simulink model "quadrotor_20181106"  (R2016a)
settings: Solver=VariableStepAuto  StartTime=t_0  StopTime=T  MaxStep=MaxStep  RelTol=RelTol  AbsTol=AbsTol
values from neighbouring files (symbols this model uses):
  J = 35000    [initialization.m]
  rule = 1    [initialization.m]
  T = 18    [initialization.m]
  x_0 = [x_0_pre;Lya_0]    [fcn_initial_uniform_eta.m]    (also in initialization.m = x_0_vec(:,i))
libraries: simulink x3
settings Model: Creator=xzbdf  LastModifiedBy=xzbdf

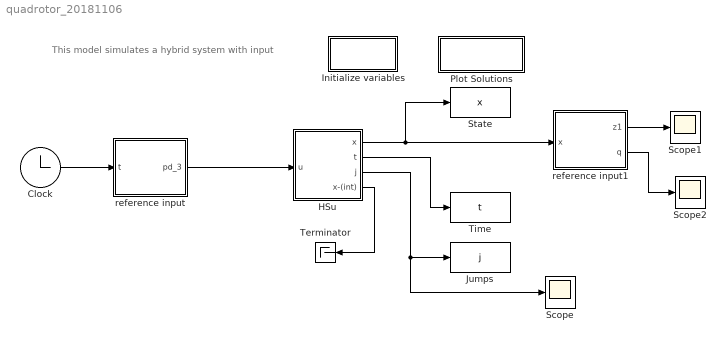
== system quadrotor_20181106 ==
  note: This model simulates a hybrid system with input
  Clock : Clock
  HSu : Subsystem  LoadFcn=set_param(gcb,'LinkStatus','none')
      settings: CopyFcn=|
      | set_param(gcb,'LinkStatus','none'),
      | set_param(gcs, 'MaxStep', 'MaxStep', 'RelTol', 'RelTol','Stop time', 'T')
      mask Display:
      | image(imread('Hcal.jpg'))
      | %plot([5 20 20 5 5],[5 5 20 20 5])
      | %text(8,13,'HyEq_mdl')
      | port_label('output', 1, 'x')
      | port_label('output', 2, 't')
      | port_label('output', 3, 'j')
      | port_label('output', 4, 'x-(int)')
      | port_label('input', 1, 'u')
  Initialize variables : Subsystem  Priority=-10
      settings: OpenFcn=|
      | try
      |      clearvars -except inifile pathfile_in pathfile_pos posfile
      |      cd(pathfile_in);
      |      eval(inifile);
      | catch
      |      [inifile,pathfile_in] = getInitializationfile;
      |      cd(pathfile_in);
      |      inifile = strrep(inifile,'.m','');
      |      eval(inifile);
      | end
      mask Display: disp('Double Click\n to Initialize')
  Jumps : ToWorkspace  VariableName=j  SampleTime=-1
      settings: Save2DSignal=2-D array (concatenate along first dimension)
  Plot Solutions : Subsystem
      settings: OpenFcn=|
      | try
      |      cd(pathfile_pos);
      |      eval(posfile);
      | catch
      |      [posfile,pathfile_pos] = getInitializationfile;
      |      cd(pathfile_pos);
      |      posfile = strrep(posfile,'.m','');
      |      eval(posfile);
      | end
      mask Display: disp('Double Click to\n Plot Solutions')
  Scope : Scope
  Scope1 : Scope
  Scope2 : Scope
  State : ToWorkspace  VariableName=x  SampleTime=-1
  Terminator : Terminator
  Time : ToWorkspace  VariableName=t  SampleTime=-1
      settings: Save2DSignal=2-D array (concatenate along first dimension)
  reference input : MATLAB Function  TreatAsAtomicUnit=on
  reference input1 : MATLAB Function  TreatAsAtomicUnit=on
  wires:
  Clock/1 -> reference input/1(t)
  reference input/1(pd_3) -> HSu/1(u)
  HSu/4(x-(int)) -> Terminator/1
  HSu/1(x) -> reference input1/1(x), State/1
  HSu/2(t) -> Time/1
  HSu/3(j) -> Scope/1, Jumps/1
  reference input1/1(z1) -> Scope1/1
  reference input1/2(q) -> Scope2/1

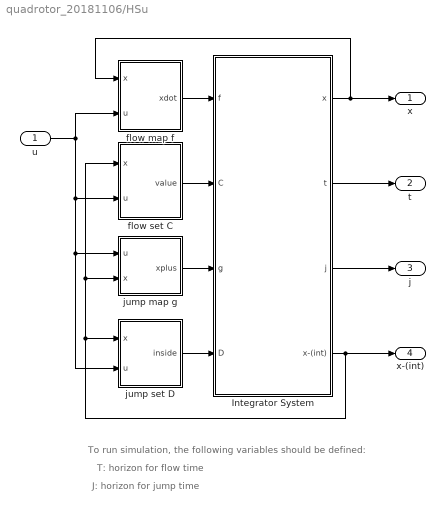
== system quadrotor_20181106/HSu ==
  note: J: horizon for jump time
  note: T: horizon for flow time
  note: To run simulation, the following variables should be defined:
  u : Inport
  Integrator System : Subsystem  Priority=2  mask(Hybrid Integrator){T=T, J=J, x0=x_0}
      mask prompts: T "Flow Horizon"; J "Jump Horizon"; x0 "Initial Condition"
      mask help:
      | This block integrates the state of the hybrid system defined by the flow map f (first input), the flow set C (second input), the jump map g (third input) and the jump set D (fourth input).
      | Starting from the initial condition x0 (last mask parameter), the system's state x evolves continuously within the set C, according to f(x,u), but is also subject to jumps within D, according to g(x,u).
      | The block also stops the simulation when the time t is greater than the flow horizon T (first mask parameter), or when the number of jumps j is greater than the jump horizon J (second mask parameter).
      | The outputs of the blocks are respectively x(t), t, j, x(t-).
      mask Help:
      | This block integrates the state of the hybrid system defined by the flow map f (first input), the flow set C (second input), the jump map g (third input) and the jump set D (fourth input).
      | <br>
      | Starting from the initial condition x0 (last mask parameter), the system's state x evolves continuously within the set C, according to f(x,u), but is also subject to jumps within D, according to g(x,u).
      | <br>
      | The block also stops the simulation when the time t is greater than the flow horizon T (first mask parameter), or when the number of jumps j is greater than the jump horizon J (second mask parameter).
      | <br>
      | The outputs of the blocks are respectively x(t), t, j, x(t-).
      | <br>
      | You can right click on the block and "Look under mask" to see what's inside the block.
      | Finally, refer to the manual (HybridSimulator_vXX.pdf) for more detailed information on how this hybrid simulator works.
  flow map f : MATLAB Function  TreatAsAtomicUnit=on
  flow set C : MATLAB Function  TreatAsAtomicUnit=on
  jump map g : MATLAB Function  Priority=2  TreatAsAtomicUnit=on
  jump set D : MATLAB Function  TreatAsAtomicUnit=on
  x : Outport
  t : Outport  Port=2
  j : Outport  Port=3
  x-(int) : Outport  Port=4
  wires:
  jump map g/1(xplus) -> Integrator System/3(g)
  jump set D/1(inside) -> Integrator System/4(D)
  u/1 -> jump set D/2(u), jump map g/1(u), flow set C/2(u), flow map f/2(u)
  Integrator System/3(j) -> j/1
  Integrator System/2(t) -> t/1
  flow set C/1(value) -> Integrator System/2(C)
  Integrator System/1(x) -> x/1, flow map f/1(x)
  Integrator System/4(x-(int)) -> x-(int)/1, flow set C/1(x), jump map g/2(x), jump set D/1(x)
  flow map f/1(xdot) -> Integrator System/1(f)

== system quadrotor_20181106/Initialize variables ==

== system quadrotor_20181106/Plot Solutions ==

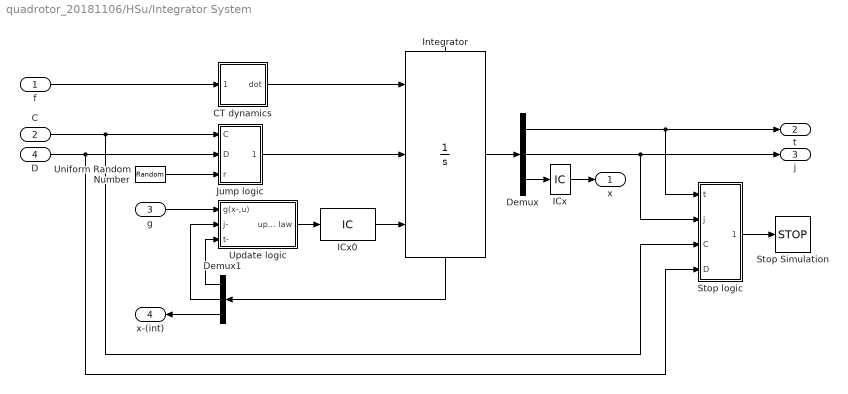
== system quadrotor_20181106/HSu/Integrator System ==
  f : Inport
  C : Inport  Port=2
  g : Inport  Port=3
  D : Inport  Port=4
  CT dynamics : Subsystem
  Demux : Demux  Outputs=[1 1 -1]
  Demux1 : Demux  Outputs=[1 1 -1]
  ICx : InitialCondition  Value=x_0
  ICx0 : InitialCondition  Value=[0; 0; x_0(:)]
  Integrator : Integrator  ExternalReset=level hold  InitialConditionSource=external  ShowStatePort=on  ZeroCross=off
  Jump logic : Subsystem
  Stop Simulation : Stop
  Stop logic : Subsystem
  Uniform Random Number : UniformRandomNumber  Minimum=0  Seed=abs(floor(100*rand))  SampleTime=0
  Update logic : Subsystem
  x : Outport
  t : Outport  Port=2
  j : Outport  Port=3
  x-(int) : Outport  Port=4
  wires:
  ICx0/1 -> Integrator/3
  ICx/1 -> x/1
  Demux/3 -> ICx/1
  Integrator/State -> Demux1/1
  Demux/2 -> j/1, Stop logic/2(j)
  Demux/1 -> t/1, Stop logic/1(t)
  Update logic/1(update law) -> ICx0/1
  CT dynamics/1(dot) -> Integrator/1
  Stop logic/1(stop) -> Stop Simulation/1
  Integrator/1 -> Demux/1
  C/1 -> Stop logic/3(C), Jump logic/1(C)
  D/1 -> Stop logic/4(D), Jump logic/2(D)
  f/1 -> CT dynamics/1(f(x,u))
  Demux1/3 -> x-(int)/1
  Jump logic/1(jump) -> Integrator/2
  Uniform Random Number/1 -> Jump logic/3(r)
  g/1 -> Update logic/1(g(x-,u))
  Demux1/1 -> Update logic/3(t-)
  Demux1/2 -> Update logic/2(j-)

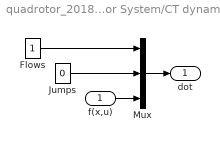
== system quadrotor_20181106/HSu/Integrator System/CT dynamics ==
  f(x,u) : Inport
  Flows : Constant
  Jumps : Constant  Value=0
  Mux : Mux  Inputs=[1 1 -1]
  dot : Outport
  wires:
  Jumps/1 -> Mux/2
  Flows/1 -> Mux/1
  Mux/1 -> dot/1
  f(x,u)/1 -> Mux/3

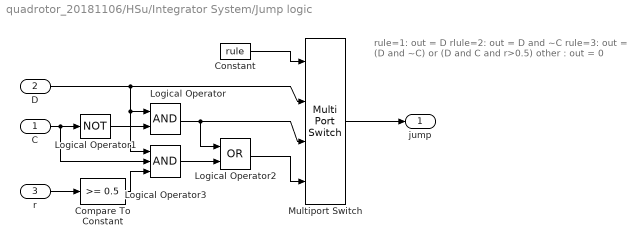
== system quadrotor_20181106/HSu/Integrator System/Jump logic ==
  note: rule=1:  out = D
      | rlule=2: out = D and ~C
      | rule=3:  out = (D and ~C)  or (D and C and r>0.5)
      | other :  out = 0
  C : Inport
  D : Inport  Port=2
  r : Inport  Port=3
  Compare To Constant : simulink/Logic and Bit Operations/Compare To Constant  relop=>=  const=0.5  OutDataTypeStr=uint8
  Constant : Constant  Value=rule
  Logical Operator : Logic  AllPortsSameDT=off  OutDataTypeStr=boolean
  Logical Operator1 : Logic  Operator=NOT  Inputs=1  AllPortsSameDT=off  OutDataTypeStr=boolean
  Logical Operator2 : Logic  Operator=OR  AllPortsSameDT=off  OutDataTypeStr=boolean
  Logical Operator3 : Logic  Inputs=3  AllPortsSameDT=off  OutDataTypeStr=boolean
  Multiport Switch : MultiPortSwitch
  jump : Outport
  wires:
  Constant/1 -> Multiport Switch/1
  D/1 -> Logical Operator3/1, Logical Operator/1, Multiport Switch/2
  r/1 -> Compare To Constant/1
  C/1 -> Logical Operator3/2, Logical Operator1/1
  Logical Operator1/1 -> Logical Operator/2
  Logical Operator/1 -> Multiport Switch/3, Logical Operator2/1
  Logical Operator2/1 -> Multiport Switch/4
  Multiport Switch/1 -> jump/1
  Compare To Constant/1 -> Logical Operator3/3
  Logical Operator3/1 -> Logical Operator2/2

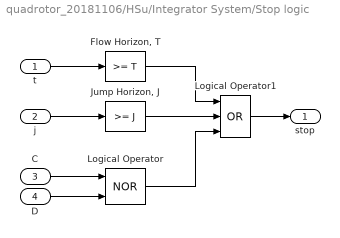
== system quadrotor_20181106/HSu/Integrator System/Stop logic ==
  t : Inport
  j : Inport  Port=2
  C : Inport  Port=3
  D : Inport  Port=4
  "Flow Horizon, T" : simulink/Logic and Bit Operations/Compare To Constant  relop=>=  const=T  OutDataTypeStr=uint8  ZeroCross=off
  "Jump Horizon, J" : simulink/Logic and Bit Operations/Compare To Constant  relop=>=  const=J  OutDataTypeStr=uint8  ZeroCross=off
  Logical Operator : Logic  Operator=NOR  AllPortsSameDT=off  OutDataTypeStr=boolean
  Logical Operator1 : Logic  Operator=OR  Inputs=3  AllPortsSameDT=off  OutDataTypeStr=boolean
  stop : Outport
  wires:
  "Flow Horizon, T"/1 -> Logical Operator1/1
  "Jump Horizon, J"/1 -> Logical Operator1/2
  Logical Operator/1 -> Logical Operator1/3
  D/1 -> Logical Operator/2
  t/1 -> "Flow Horizon, T"/1
  j/1 -> "Jump Horizon, J"/1
  C/1 -> Logical Operator/1
  Logical Operator1/1 -> stop/1

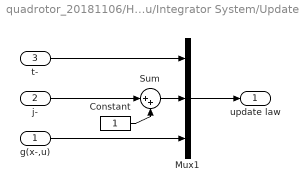
== system quadrotor_20181106/HSu/Integrator System/Update logic ==
  g(x-,u) : Inport
  j- : Inport  Port=2
  t- : Inport  Port=3
  Constant : Constant
  Mux1 : Mux  Inputs=[1 1 -1]
  Sum : Sum  Inputs=|++
  update law : Outport
  wires:
  Sum/1 -> Mux1/2
  Mux1/1 -> update law/1
  j-/1 -> Sum/1
  g(x-,u)/1 -> Mux1/3
  t-/1 -> Mux1/1
  Constant/1 -> Sum/2

== matlab function quadrotor_20181106/reference input1 ==
  data: z1 output; x input; q output
function [z1,q]=fcn_z1(x)

z1=x(10:12);
q=x(23);

end

== matlab function quadrotor_20181106/reference input ==
  data: pd_3 output; t input; para parameter
function pd_3 = fcn_pd_3(t, para)

r_index=para(1);
m=para(2);
gra=para(3);
k1=para(4);
k2=para(5);
gamma=para(6);
kw=para(7);
M_beta=para(8);
K_beta=para(9);
e1=para(10:12);
e2=para(13:15);
e3=para(16:18);
epsilon=para(19);
sigma=para(20);


if r_index==1
        [~,~,~,pd_3] = r_circle(t);
elseif r_index==2
        [~,~,~,pd_3] = r_lemniscate(t);
else 
        [~,~,~,pd_3] = r_stationary(t);
end

% switch r_index
%     case 1
%         [~,~,~,pd_3] = r_circle(t);
%     case 2
%         [~,~,~,pd_3] = r_lemniscate(t);
%     case 3
%         [~,~,~,pd_3] = r_stationary(t);
% end

end

== matlab function quadrotor_20181106/HSu/flow map f ==
  data: x input; xdot output; u input; para parameter
function xdot = f(x,u,para)

m=para(2);
gra=para(3);
e3=para(16:18);

pd_1=x(4:6);
pd_2=x(7:9);
z2=x(13:15);
r3=x(16:18);
s1=x(19);
s2=x(20:22);

pd_3=u;

pdd=pd_1;
pd_1d=pd_2;
pd_2d=pd_3;

z1d=z2;
z2d=-1./m.*r3*s1+gra.*e3-pd_2;
r3d=-S(r3)*s2;

s1d=0;
s2d=zeros(3,1);
qd=0;

f_map=[pdd;pd_1d;pd_2d;z1d;z2d;r3d;s1d;s2d;qd];
grad_V=fcn_grad_V(x,para);

Lyad=grad_V'*f_map;

xdot=[pdd;pd_1d;pd_2d;z1d;z2d;r3d;s1d;s2d;qd;Lyad];

end

== matlab function quadrotor_20181106/HSu/flow set C ==
  data: x input; value output; u input; para parameter
function value  = C(x,u,para)

m=para(2);
gra=para(3);
e3=para(16:18);
sigma=para(20);
eta=para(21);

pd=x(1:3);
pd_1=x(4:6);
pd_2=x(7:9);
z1=x(10:12);
z2=x(13:15);
r3=x(16:18);
s1=x(19);
s2=x(20:22);
xi=x(1:22);
q=x(23);

r=[pd;pd_1;pd_2];
z=[z1;z2;r3];

pd_3=u;

pdd=pd_1;
pd_1d=pd_2;
pd_2d=pd_3;
z1d=z2;
z2d=-1./m.*r3*s1+gra.*e3-pd_2;
r3d=-S(r3)*s2;
s1d=0;
s2d=zeros(3,1);
qd=0;

z2cld=-1./m.*r3*fcn_T(r,z,para)+gra.*e3-pd_2;
r3cld=-S(r3)*fcn_w(r,z,pd_3,q,para);

f_map=[pdd;pd_1d;pd_2d;z1d;z2d;r3d;s1d;s2d;qd];
fcl_map=[pdd;pd_1d;pd_2d;z1d;z2cld;r3cld;s1d;s2d;qd];

grad_V=fcn_grad_V(x,para);

% if (grad_Vq'*f<=sigma.*Lyacldot)%not correct, because there are numerical errors
% due to the equation I_3-r3^\top*r3=-S^2(r3) when getting the closed-loop
% expression for eqn 12
%%%C_1\cap C_2
value_C_1=(fcn_V(x,para)-min(fcn_V([xi;-1],para),fcn_V([xi;1],para))<=eta);
value_C_2=(grad_V'*f_map<=sigma.*grad_V'*fcl_map);
if (value_C_1==1)&&(value_C_2==1)
    value = 1;
else
    value = 0;
end


end

== matlab function quadrotor_20181106/HSu/jump map g ==
  data: xplus output; u input; para parameter; x input
function xplus = g(u,para, x)

m=para(2);
gra=para(3);
e3=para(16:18);
epsilon=para(19);
sigma=para(20);
eta=para(21);

pd=x(1:3);
pd_1=x(4:6);
pd_2=x(7:9);
z1=x(10:12);
z2=x(13:15);
r3=x(16:18);
s1=x(19);
s2=x(20:22);
xi=x(1:22);
q=x(23);
Lya=x(24);
r=[pd;pd_1;pd_2];
z=[z1;z2;r3];
zeta=[r;z1;z2];

pd_3=u;

pdplus=pd;
pd_1plus=pd_1;
pd_2plus=pd_2;
z1plus=z1;
z2plus=z2;
r3plus=r3;

%%%%%%%%%%%%%%%%%%%%%%%%%%%%
pdd=pd_1;
pd_1d=pd_2;
pd_2d=pd_3;
z1d=z2;
z2d=-1./m.*r3*s1+gra.*e3-pd_2;
r3d=-S(r3)*s2;
s1d=0;
s2d=zeros(3,1);
qd=0;

z2cld=-1./m.*r3*fcn_T(r,z,para)+gra.*e3-pd_2;
r3cld=-S(r3)*fcn_w(r,z,pd_3,q,para);

f_map=[pdd;pd_1d;pd_2d;z1d;z2d;r3d;s1d;s2d;qd];
fcl_map=[pdd;pd_1d;pd_2d;z1d;z2cld;r3cld;s1d;s2d;qd];

grad_V=fcn_grad_V(x,para);

inside_D_1=(fcn_V(x,para)-min(fcn_V([xi;-1],para),fcn_V([xi;1],para))>=eta);
inside_D_2=(grad_V'*f_map>=sigma.*grad_V'*fcl_map);
%%%in D_1, not in D_2
if (inside_D_1==1)&&(inside_D_2==0)
    s1plus=s1;
    s2plus=s2;
    qplus=-q;
    Lyaplus=Lya+2.*epsilon.*q.*r3'*fcn_r3d(zeta,para);

%%%in D_2, not in D_1
elseif (inside_D_2==1)&&(inside_D_1==0)
    s1plus=fcn_T(r,z,para);
    s2plus=fcn_w(r,z,pd_3,q,para);
    qplus=q;
    Lyaplus=Lya;

%%%in D_1\cap D_2: (inside_D_2==1)&&(inside_D_1==1)
else 
    Random_index=round(rand(1));%%%%%%%%%%notice!!!!!!!!!!! (s1, s2, -q) OR (T,w,q)
    possible_s1plus=[s1,fcn_T(r,z,para)];
    s1plus=possible_s1plus(Random_index+1);
    possible_s2plus=[s2,fcn_w(r,z,pd_3,q,para)];
    s2plus=possible_s2plus(:,Random_index+1);
    qplus=(-1)^(Random_index+1).*q;
    
    if qplus==q
        Lyaplus=Lya; 
%%% qplus==(-q)
    else
        Lyaplus=Lya+2.*epsilon.*q.*r3'*fcn_r3d(zeta,para);
    end
end
%%%%%%%%%%%%%%%%%%%%%%%%%%%%%%%%%%%%%%%%%%%
xplus=[pdplus;pd_1plus;pd_2plus;z1plus;z2plus;r3plus;s1plus;s2plus;qplus;Lyaplus];

end

== matlab function quadrotor_20181106/HSu/jump set D ==
  data: x input; inside output; u input; para parameter
function inside  = D(x,u,para)

m=para(2);
gra=para(3);
e3=para(16:18);
sigma=para(20);
eta=para(21);

pd=x(1:3);
pd_1=x(4:6);
pd_2=x(7:9);
z1=x(10:12);
z2=x(13:15);
r3=x(16:18);
s1=x(19);
s2=x(20:22);
xi=x(1:22);
q=x(23);

r=[pd;pd_1;pd_2];
z=[z1;z2;r3];

pd_3=u;

pdd=pd_1;
pd_1d=pd_2;
pd_2d=pd_3;
z1d=z2;
z2d=-1./m.*r3*s1+gra.*e3-pd_2;
r3d=-S(r3)*s2;
s1d=0;
s2d=zeros(3,1);
qd=0;

z2cld=-1./m.*r3*fcn_T(r,z,para)+gra.*e3-pd_2;
r3cld=-S(r3)*fcn_w(r,z,pd_3,q,para);

f_map=[pdd;pd_1d;pd_2d;z1d;z2d;r3d;s1d;s2d;qd];
fcl_map=[pdd;pd_1d;pd_2d;z1d;z2cld;r3cld;s1d;s2d;qd];

grad_V=fcn_grad_V(x,para);

%%%D_1\cup D_2
inside_D_1=(fcn_V(x,para)-min(fcn_V([xi;-1],para),fcn_V([xi;1],para))>=eta);
inside_D_2=(grad_V'*f_map>=sigma.*grad_V'*fcl_map);
if (inside_D_1==1)||(inside_D_2==1)
    inside = 1;
else
    inside = 0;
end

end
